simulink model "PC_tmp"  (R2021b)
settings: Solver=FixedStepAuto  StartTime=0.0  StopTime=100  RelTol=1e-3
settings Model: Creator=kboxi  LastModifiedBy=kboxi

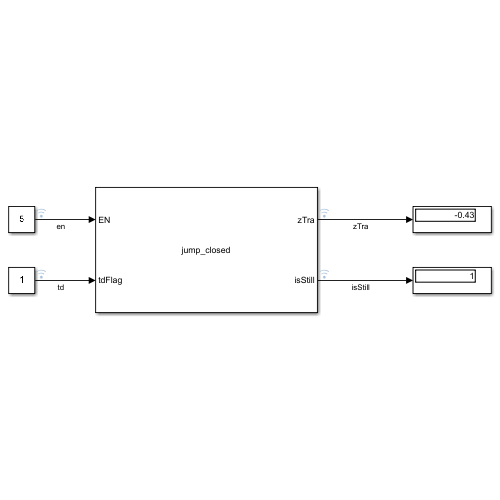
[thumbnail: Simulink's stored preview of the top-level diagram]
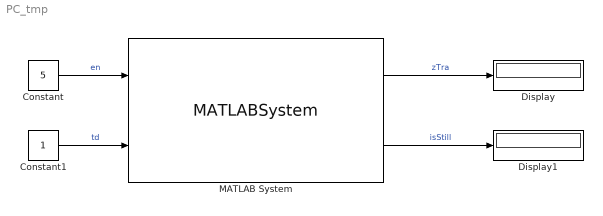
== system PC_tmp ==
  Constant : Constant  Value=5
  Constant1 : Constant
  Display : Display
  Display1 : Display
  MATLAB System : MATLABSystem  System=jump_closed  tsk=0.15  tst=0.05  tst_wt=0.1  tdy=0.05  lh=0.07  zOff=-0.5  SampleTime=0.004  OffsetTime=0  TickTime=0  SimulateUsing=Code generation
      mask Type: jump_closed
      mask Display:
      | disp('jump_closed');
      | port_label('input',1,'EN');
      | port_label('input',2,'tdFlag');
      | port_label('output',1,'zTra');
      | port_label('output',2,'isStill');
  wires:
  MATLAB System/1 -> Display/1  "zTra"
  MATLAB System/2 -> Display1/1  "isStill"
  Constant/1 -> MATLAB System/1  "en"
  Constant1/1 -> MATLAB System/2  "td"
